simulink model "Simscape_Benchmark_SIM1"  (R2021a)
settings: Solver=ode45  StartTime=0.0  StopTime=PHASE.Ttotal  FixedStep=Benchmark.Sim.Tint  RelTol=1e-5  AbsTol=1e-6
undefined symbols (not defined in the file): Actuators, Analysis, antisym, Benchmark, Bus, Disturbance, FSM, IntialCond, ISOL, K_Coarse_disc_t, Kslew_opt_disc_zoh, Model, MPS, PAYLOAD, PHASE, PMA, RWIsol, RWS, SA, Sensors, Slew, slosh, thr, X, Y, Z
libraries: sm_lib x215, nesl_utility x148, simulink x65, cstblocks x36, sharedtransform x4, vrlib x3, RCTblocks x1
(part 8 of 9)

== system Simscape_Benchmark_SIM1/Dynamical system/Payload System (Telescope structure, FSM, PMA system, Isolator)/Transformation sensors ==
  Mux14 : Mux  Inputs=2
  Mux{15..16,20..21} (4 alike) : Mux  Inputs=3
  Mux22 : Mux  Inputs=2
  PS-Simulink Converter{13..15,40..48} (12 alike) : nesl_utility/PS-Simulink Converter  PhysicalDomain=network_engine_domain  SubClassName=ps_output  LeftPortType=input  RightPortType=output  PseudoPeriodic=off  Frequencies=[]  Unit=inherit  AffineConversion=off
      settings: SourceProductBaseCode=PW,SS
  Transform Sensor4 : sm_lib/Frames and Transforms/Transform Sensor  MeasurementFrame=NonRotatingFollower  SenseAngle=off  SenseAxis=off  SenseAngle1=off  SenseAngle2=off  SenseAngle3=off  SenseQ=off  SenseR=off  SenseOmegaX=off  SenseOmegaY=off  SenseOmegaZ=off  SenseOmega1=off  SenseOmega2=off  SenseOmega3=off  SenseQDot=off  SenseRDot=off  SenseAlphaX=on  SenseAlphaY=on  SenseAlphaZ=on  SenseAlpha1=off  SenseAlpha2=off  SenseAlpha3=off  SenseQDDot=off  SenseRDDot=off  SenseX=off  SenseY=off  SenseZ=off  SenseRad=off  SenseAzim=off  SenseDist=off  SenseInc=off  SenseXDot=off  SenseYDot=off  SenseZDot=off  SenseRadDot=off  SenseAzimDot=off  SenseDistDot=off  SenseIncDot=off  SenseXDDot=on  SenseYDDot=on  SenseZDDot=on  SenseRadDDot=off  SenseAzimDDot=off  SenseDistDDot=off  SenseIncDDot=off
  Transform Sensor7 : sm_lib/Frames and Transforms/Transform Sensor  MeasurementFrame=Base  SenseAngle=off  SenseAxis=off  SenseAngle1=off  SenseAngle2=off  SenseAngle3=off  SenseQ=off  SenseR=off  SenseOmegaX=off  SenseOmegaY=off  SenseOmegaZ=off  SenseOmega1=off  SenseOmega2=off  SenseOmega3=off  SenseQDot=off  SenseRDot=off  SenseAlphaX=on  SenseAlphaY=on  SenseAlphaZ=on  SenseAlpha1=off  SenseAlpha2=off  SenseAlpha3=off  SenseQDDot=off  SenseRDDot=off  SenseX=off  SenseY=off  SenseZ=off  SenseRad=off  SenseAzim=off  SenseDist=off  SenseInc=off  SenseXDot=off  SenseYDot=off  SenseZDot=off  SenseRadDot=off  SenseAzimDot=off  SenseDistDot=off  SenseIncDot=off  SenseXDDot=on  SenseYDDot=on  SenseZDDot=on  SenseRadDDot=off  SenseAzimDDot=off  SenseDistDDot=off  SenseIncDDot=off
  Transform Sensor1 : PMIOPort  Side=Left
  Transform Sensor2 : PMIOPort  Port=2  Side=Left
  xdd_MPC_nonrotating : Outport
  xdd_MPC_Inertial : Outport  Port=2
  wires:
  PS-Simulink Converter45/1 -> Mux15/1
  Mux21/1 -> Mux22/1
  PS-Simulink Converter44/1 -> Mux16/3
  PS-Simulink Converter46/1 -> Mux15/2
  PS-Simulink Converter41/1 -> Mux20/2
  Mux15/1 -> Mux14/2
  PS-Simulink Converter43/1 -> Mux16/2
  Mux14/1 -> xdd_MPC_nonrotating/1
  PS-Simulink Converter48/1 -> Mux20/3
  PS-Simulink Converter47/1 -> Mux15/3
  Mux16/1 -> Mux14/1
  PS-Simulink Converter40/1 -> Mux20/1
  PS-Simulink Converter15/1 -> Mux21/3
  PS-Simulink Converter13/1 -> Mux21/1
  PS-Simulink Converter14/1 -> Mux21/2
  PS-Simulink Converter42/1 -> Mux16/1
  Mux20/1 -> Mux22/2
  Mux22/1 -> xdd_MPC_Inertial/1  "xdd_MPC_Inertial"
  connections:
  Transform Sensor7/RConn1 -- Transform Sensor2/RConn1 -- Transform Sensor4/RConn1
  Transform Sensor4/RConn7 -- PS-Simulink Converter44/LConn1
  Transform Sensor7/LConn1 -- Transform Sensor1/RConn1 -- Transform Sensor4/LConn1
  Transform Sensor4/RConn2 -- PS-Simulink Converter45/LConn1
  Transform Sensor7/RConn6 -- PS-Simulink Converter14/LConn1
  Transform Sensor7/RConn2 -- PS-Simulink Converter40/LConn1
  Transform Sensor4/RConn6 -- PS-Simulink Converter43/LConn1
  Transform Sensor4/RConn3 -- PS-Simulink Converter46/LConn1
  Transform Sensor7/RConn5 -- PS-Simulink Converter13/LConn1
  Transform Sensor4/RConn5 -- PS-Simulink Converter42/LConn1
  Transform Sensor7/RConn3 -- PS-Simulink Converter41/LConn1
  Transform Sensor7/RConn4 -- PS-Simulink Converter48/LConn1
  Transform Sensor7/RConn7 -- PS-Simulink Converter15/LConn1
  Transform Sensor4/RConn4 -- PS-Simulink Converter47/LConn1

== system Simscape_Benchmark_SIM1/Dynamical system/Payload System (Telescope structure, FSM, PMA system, Isolator)/Transformation sensors 2 ==
  Mux13 : Mux  Inputs=2
  Mux2 : Mux  Inputs=3
  Mux3 : Mux  Inputs=3
  PS-Simulink Converter{18..23} (6 alike) : nesl_utility/PS-Simulink Converter  PhysicalDomain=network_engine_domain  SubClassName=ps_output  LeftPortType=input  RightPortType=output  PseudoPeriodic=off  Frequencies=[]  Unit=inherit  AffineConversion=off
      settings: SourceProductBaseCode=PW,SS
  Transform Sensor3 : sm_lib/Frames and Transforms/Transform Sensor  MeasurementFrame=Base  SenseAngle=off  SenseAxis=off  SenseAngle1=off  SenseAngle2=off  SenseAngle3=off  SenseQ=off  SenseR=off  SenseOmegaX=off  SenseOmegaY=off  SenseOmegaZ=off  SenseOmega1=off  SenseOmega2=off  SenseOmega3=off  SenseQDot=off  SenseRDot=off  SenseAlphaX=on  SenseAlphaY=on  SenseAlphaZ=on  SenseAlpha1=off  SenseAlpha2=off  SenseAlpha3=off  SenseQDDot=off  SenseRDDot=off  SenseX=off  SenseY=off  SenseZ=off  SenseRad=off  SenseAzim=off  SenseDist=off  SenseInc=off  SenseXDot=off  SenseYDot=off  SenseZDot=off  SenseRadDot=off  SenseAzimDot=off  SenseDistDot=off  SenseIncDot=off  SenseXDDot=on  SenseYDDot=on  SenseZDDot=on  SenseRadDDot=off  SenseAzimDDot=off  SenseDistDDot=off  SenseIncDDot=off
  Transform Sensor2 : PMIOPort  Side=Left
  Transform Sensor1 : PMIOPort  Port=2  Side=Left
  Out1 : Outport
  wires:
  PS-Simulink Converter19/1 -> Mux3/2
  PS-Simulink Converter18/1 -> Mux3/1
  Mux3/1 -> Mux13/1
  Mux13/1 -> Out1/1
  Mux2/1 -> Mux13/2
  PS-Simulink Converter21/1 -> Mux2/1
  PS-Simulink Converter22/1 -> Mux2/2
  PS-Simulink Converter20/1 -> Mux3/3
  PS-Simulink Converter23/1 -> Mux2/3
  connections:
  PS-Simulink Converter20/LConn1 -- Transform Sensor3/RConn7
  Transform Sensor3/RConn5 -- PS-Simulink Converter18/LConn1
  Transform Sensor3/RConn4 -- PS-Simulink Converter23/LConn1
  Transform Sensor3/RConn3 -- PS-Simulink Converter22/LConn1
  Transform Sensor3/RConn2 -- PS-Simulink Converter21/LConn1
  Transform Sensor3/RConn6 -- PS-Simulink Converter19/LConn1
  Transform Sensor2/RConn1 -- Transform Sensor3/LConn1
  Transform Sensor3/RConn1 -- Transform Sensor1/RConn1

== system Simscape_Benchmark_SIM1/Dynamical system/RCS models/RCS (thruster model) ==
  Cmd_force : Inport  PortDimensions=3
  Cmd_Torque : Inport  Port=2  PortDimensions=3
  Allocation Function (Updated) : MATLABFcn  MATLABFcn=Thr_AllocationFunct  OutputDimensions=thr.nb_thr+1
  Clock : Clock
  Constant : Constant  Value=thr.sc_thrust_Ht
  Constant1 : Constant  Value=thr.F
  Constant10 : Constant  Value=thr.sc_thrust_Ht_reshaped'
  Constant11 : Constant  Value=thr.nb_thr
  Constant13 : Constant  Value=thr.F
  Constant2 : Constant  Value=thr.sc_thrust_Hf
  Constant3 : Constant  Value=thr.nb_thr
  Constant4 : Constant  Value=Model.ACS_sampling.Ts
  Constant6 : Constant  Value=thr.u_min
  Constant8 : Constant  Value=zeros(thr.nb_thr,1)
  Constant9 : Constant  Value=thr.sc_thrust_Hf_reshaped'
  Demux1 : Demux  Outputs=[thr.nb_thr,1]
  Demux2 : Demux  Outputs=[3,3]
  Gain : Gain  Gain=thr.F
  Gain1 : Gain  Gain=thr.F
  Gain2 : Gain  Gain=thr.F
  MATLAB Function1 : MATLAB Function  TreatAsAtomicUnit=on  SystemSampleTime=thr.MIB_time
  Matrix Concatenate : Concatenate  Mode=Multidimensional array
  Mux : Mux  Inputs=2
  Mux2 : Mux  Inputs=2
  Mux3 : Mux  Inputs=[6,1,1,thr.nb_thr*3,thr.nb_thr*3]
  Product : Product  Multiplication=Matrix(*)
  Scope1 : Scope  NumInputPorts=2
  Scope2 : Scope
  Sum : Sum  Inputs=-+
  Thruster dynamic response (2nd order) : cstblocks/LTI System  Commented=through  sys=tf(thr.om^2,[1 2*thr.damp*thr.om thr.om^2])*eye(thr.nb_thr)  IC=[]
  Thr_Force : Outport
  Thr_Force_NoPWM : Outport  Port=2
  Thr_activated : Outport  Port=3
  wires:
  Constant10/1 -> Mux3/5  "thr.nb_thr*3"
  Constant9/1 -> Mux3/4  "thr.nb_thr*3"
  Constant2/1 -> Matrix Concatenate/1
  Constant1/1 -> MATLAB Function1/2(u_thr)
  Constant8/1 -> MATLAB Function1/7(y_size)
  Constant3/1 -> MATLAB Function1/5(nb_thr)
  Mux2/1 -> Mux3/1, Sum/1
  Constant4/1 -> MATLAB Function1/3(Sampling_time)
  Sum/1 -> Scope2/1
  Constant/1 -> Matrix Concatenate/2
  Constant13/1 -> Mux3/3  "1"
  Demux1/1 -> Mux/2, Gain2/1, Gain/1, Product/2  "U_cont"
  Demux1/2 -> Thr_activated/1  "n_activated"
  Constant6/1 -> MATLAB Function1/4(u_min)
  Matrix Concatenate/1 -> Product/1
  Mux3/1 -> Mux/1
  Allocation Function (Updated)/1 -> Demux1/1
  Constant11/1 -> Mux3/2  "1"
  Cmd_force/1 -> Mux2/1
  Cmd_Torque/1 -> Mux2/2
  MATLAB Function1/1(y) -> Thruster dynamic response (2nd order)/1
  Clock/1 -> MATLAB Function1/6(Time)
  Demux2/1 -> Scope1/1
  Product/1 -> Sum/2, Gain1/1
  Demux2/2 -> Scope1/2
  Gain/1 -> Thr_Force_NoPWM/1
  Gain1/1 -> Demux2/1
  Mux/1 -> Allocation Function (Updated)/1
  Thruster dynamic response (2nd order)/1 -> Thr_Force/1
  Gain2/1 -> MATLAB Function1/1(U_cont)

== system Simscape_Benchmark_SIM1/Dynamical system/WEMS + Reaction wheels/Friction compensation filter ==
  speed : Inport
  torque : Inport  Port=2
  Enable : EnablePort
  1/Ts : Gain  Gain=1/Model.ACS_sampling.Ts
  Clock : Clock
  Constant : Constant  Value=0
  Constant1 : Constant  Value=[0;0;0;0]
  Delay1 : Delay  DelayLength=1  InitialConditionSource=Input port  InitialCondition=RWS.w1simscape
      settings: InputPortMap=u0,p4
  Delay2 : Delay  DelayLength=1  InitialConditionSource=Input port  InitialCondition=RWS.w2simscape
      settings: InputPortMap=u0,p4
  Delay3 : Delay  DelayLength=1  InitialCondition=0
  Delay4 : Delay  DelayLength=1  InitialConditionSource=Input port  InitialCondition=RWS.w3simscape
      settings: InputPortMap=u0,p4
  Delay5 : Delay  DelayLength=1  InitialConditionSource=Input port  InitialCondition=RWS.w4simscape
      settings: InputPortMap=u0,p4
  Demux6 : Demux
  I_wheel : Gain  Gain=RWS.Iw
  InitialCond_1 : Constant  Value=RWS.w1simscape
  InitialCond_2 : Constant  Value=RWS.w2simscape
  InitialCond_3 : Constant  Value=RWS.w3simscape
  InitialCond_4 : Constant  Value=RWS.w4simscape
  LTI System1 : cstblocks/LTI System  sys=RWS.FrictionEstimation.FilterD  IC=0
  Mux4 : Mux
  RWS.FrictionEstimation.T_excludeTransient : Constant  Value=RWS.FrictionEstimation.T_excludeTransient
  Rate Transition : RateTransition  OutPortSampleTime=Model.ACS_sampling.Ts
  Sum : Sum  Inputs=|+-
  Sum1 : Sum  Inputs=+|-
  Sum2 : Sum  Inputs=|+-
  Switch : Switch  Criteria=u2 > Threshold
  Terminator : Terminator
  Out1 : Outport  InitialOutput=[0;0;0;0]
  wires:
  Sum1/1 -> LTI System1/1
  Demux6/1 -> Delay1/1
  Constant1/1 -> Switch/3
  Delay4/1 -> Mux4/3
  Clock/1 -> Sum2/1
  Delay3/1 -> Sum1/2
  LTI System1/1 -> Switch/1
  Sum/1 -> I_wheel/1
  Switch/1 -> Out1/1  "estimated"
  Demux6/3 -> Delay4/1
  Delay2/1 -> Mux4/2
  torque/1 -> Delay3/1
  Demux6/4 -> Delay5/1
  speed/1 -> Sum/1, Demux6/1
  Delay5/1 -> Mux4/4
  Mux4/1 -> Sum/2
  Demux6/2 -> Delay2/1
  1/Ts/1 -> Sum1/1
  Rate Transition/1 -> Switch/2
  Delay1/1 -> Mux4/1
  Constant/1 -> Sum2/2
  Sum2/1 -> Rate Transition/1
  RWS.FrictionEstimation.T_excludeTransient/1 -> Terminator/1
  I_wheel/1 -> 1/Ts/1
  InitialCond_1/1 -> Delay1/2
  InitialCond_2/1 -> Delay2/2
  InitialCond_3/1 -> Delay4/2
  InitialCond_4/1 -> Delay5/2

== system Simscape_Benchmark_SIM1/Dynamical system/WEMS + Reaction wheels/RW saturation and friction model ==
  note: 1) Add Subsystem or Model blocks as valid variant choices.
      | 2) You cannot connect blocks at this level. At simulation, connectivity is automatically
      | determined, based on the active variant and port name matching.
  In1 : Inport
  No saturations - No friction model : Subsystem  VariantControl=Benchmark.config.status.RWS_Sat==0 && Benchmark.config.status.RWS_Fric==0 && Benchmark.config.status.RWS_Frict_spikes==0
  Saturations +  friction model : Subsystem  VariantControl=Benchmark.config.status.RWS_Sat==1 && Benchmark.config.status.RWS_Fric==1 && Benchmark.config.status.RWS_Frict_spikes==0
  Saturations + friction model + friction spikes : Subsystem  VariantControl=Benchmark.config.status.RWS_Sat==1 && Benchmark.config.status.RWS_Fric==1 && Benchmark.config.status.RWS_Frict_spikes==1
  Saturations - No friction model : Subsystem  VariantControl=Benchmark.config.status.RWS_Sat==1 && Benchmark.config.status.RWS_Fric==0 && Benchmark.config.status.RWS_Frict_spikes==0
  Out1 : Outport

== system Simscape_Benchmark_SIM1/Dynamical system/WEMS + Reaction wheels/Reaction wheel Mass//inertia (balanced and unbalanced model) ==
  Balanced RWS : Subsystem  VariantControl="Benchmark.config.status.RWS_Harmdist==   0"
  RWS with disturbance harmonics : Subsystem  VariantControl="Benchmark.config.status.RWS_Harmdist==   1"
  Connection Port : PMIOPort  Tag=PMCPort  Side=Left
  Connection Port1 : PMIOPort  Tag=PMCPort  Port=2  Side=Left
  Connection Port2 : PMIOPort  Tag=PMCPort  Port=3  Side=Left
  Connection Port3 : PMIOPort  Tag=PMCPort  Port=4  Side=Left

== system Simscape_Benchmark_SIM1/Sensors/Accelerometer Mirror 1/acc_M1 ==
  note: Constant PSD such that
      | its integral (from 0 to Nyquist frequency) is 1
  note: After scaling: One-sided PSD with value equal to 1
      | up to Nyquist frequency
  Gain : Gain
  Gain1 : Gain  Gain=sqrt(0.5/Sensors.ACCm1.SampleTime)
  Gain2 : Gain  Gain=sqrt(0.5/Sensors.ACCm1.SampleTime)
  Gain3 : Gain
  Gain4 : Gain
  Gain7 : Gain  Gain=sqrt(0.5/Sensors.ACCm1.SampleTime)
  Mux : Mux  Inputs=6
  Noise_accM1_rotx : simulink/Sources/Band-Limited White Noise  Cov=Sensors.ACCm1.NoiseProtx  Ts=Sensors.ACCm1.SampleTime  seed=Sensors.ACCm1.Seed(4)
  Noise_accM1_roty : simulink/Sources/Band-Limited White Noise  Cov=Sensors.ACCm1.NoiseProty  Ts=Sensors.ACCm1.SampleTime  seed=Sensors.ACCm1.Seed(5)
  Noise_accM1_rotz : simulink/Sources/Band-Limited White Noise  Cov=Sensors.ACCm1.NoiseProtz  Ts=Sensors.ACCm1.SampleTime  seed=Sensors.ACCm1.Seed(6)
  Noise_accM1_x : simulink/Sources/Band-Limited White Noise  Cov=Sensors.ACCm1.NoisePx  Ts=Sensors.ACCm1.SampleTime  seed=Sensors.ACCm1.Seed(1)
  Noise_accM1_y : simulink/Sources/Band-Limited White Noise  Cov=Sensors.ACCm1.NoisePy  Ts=Sensors.ACCm1.SampleTime  seed=Sensors.ACCm1.Seed(2)
  Noise_accM1_z : simulink/Sources/Band-Limited White Noise  Cov=Sensors.ACCm1.NoisePz  Ts=Sensors.ACCm1.SampleTime  seed=Sensors.ACCm1.Seed(3)
  Sensors.ACCm1.NoisePxFilter : cstblocks/LTI System  sys=Sensors.ACCm1.NoisePxFilter  IC=[]
  Sensors.ACCm1.NoisePyFilter : cstblocks/LTI System  sys=Sensors.ACCm1.NoisePyFilter  IC=[]
  Sensors.ACCm1.NoisePzFilter : cstblocks/LTI System  sys=Sensors.ACCm1.NoisePzFilter  IC=[]
  Out1 : Outport
  wires:
  Sensors.ACCm1.NoisePxFilter/1 -> Mux/1
  Mux/1 -> Out1/1
  Gain1/1 -> Sensors.ACCm1.NoisePyFilter/1
  Gain7/1 -> Sensors.ACCm1.NoisePxFilter/1
  Sensors.ACCm1.NoisePyFilter/1 -> Mux/2
  Sensors.ACCm1.NoisePzFilter/1 -> Mux/3
  Noise_accM1_rotx/1 -> Gain/1
  Noise_accM1_roty/1 -> Gain3/1
  Noise_accM1_rotz/1 -> Gain4/1
  Noise_accM1_x/1 -> Gain7/1
  Noise_accM1_y/1 -> Gain1/1
  Noise_accM1_z/1 -> Gain2/1
  Gain2/1 -> Sensors.ACCm1.NoisePzFilter/1
  Gain/1 -> Mux/4
  Gain3/1 -> Mux/5
  Gain4/1 -> Mux/6

== system Simscape_Benchmark_SIM1/Sensors/Accelerometer Mirror 2/acc_M2 ==
  Gain1 : Gain  Gain=sqrt(0.5/Sensors.ACCm2.SampleTime)
  Gain2 : Gain  Gain=sqrt(0.5/Sensors.ACCm2.SampleTime)
  Gain3 : Gain
  Gain4 : Gain
  Gain5 : Gain
  Gain7 : Gain  Gain=sqrt(0.5/Sensors.ACCm2.SampleTime)
  Mux : Mux  Inputs=6
  Noise_accM2_rotx : simulink/Sources/Band-Limited White Noise  Cov=Sensors.ACCm2.NoiseProtx  Ts=Sensors.ACCm2.SampleTime  seed=Sensors.ACCm2.Seed(4)
  Noise_accM2_roty : simulink/Sources/Band-Limited White Noise  Cov=Sensors.ACCm2.NoiseProty  Ts=Sensors.ACCm2.SampleTime  seed=Sensors.ACCm2.Seed(5)
  Noise_accM2_rotz : simulink/Sources/Band-Limited White Noise  Cov=Sensors.ACCm2.NoiseProtz  Ts=Sensors.ACCm2.SampleTime  seed=Sensors.ACCm2.Seed(6)
  Noise_accM2_x : simulink/Sources/Band-Limited White Noise  Cov=Sensors.ACCm2.NoisePx  Ts=Sensors.ACCm2.SampleTime  seed=Sensors.ACCm2.Seed(1)
  Noise_accM2_y : simulink/Sources/Band-Limited White Noise  Cov=Sensors.ACCm2.NoisePy  Ts=Sensors.ACCm2.SampleTime  seed=Sensors.ACCm2.Seed(2)
  Noise_accM2_z : simulink/Sources/Band-Limited White Noise  Cov=Sensors.ACCm2.NoisePz  Ts=Sensors.ACCm2.SampleTime  seed=Sensors.ACCm2.Seed(3)
  Sensors.ACCm2.NoisePxFilter : cstblocks/LTI System  sys=Sensors.ACCm2.NoisePxFilter  IC=[]
  Sensors.ACCm2.NoisePyFilter : cstblocks/LTI System  sys=Sensors.ACCm2.NoisePyFilter  IC=[]
  Sensors.ACCm2.NoisePzFilter : cstblocks/LTI System  sys=Sensors.ACCm2.NoisePzFilter  IC=[]
  Out1 : Outport
  wires:
  Sensors.ACCm2.NoisePxFilter/1 -> Mux/1
  Mux/1 -> Out1/1
  Gain1/1 -> Sensors.ACCm2.NoisePyFilter/1
  Gain2/1 -> Sensors.ACCm2.NoisePzFilter/1
  Gain7/1 -> Sensors.ACCm2.NoisePxFilter/1
  Sensors.ACCm2.NoisePyFilter/1 -> Mux/2
  Sensors.ACCm2.NoisePzFilter/1 -> Mux/3
  Noise_accM2_rotz/1 -> Gain5/1
  Gain3/1 -> Mux/4
  Gain4/1 -> Mux/5
  Noise_accM2_z/1 -> Gain2/1
  Noise_accM2_y/1 -> Gain1/1
  Noise_accM2_x/1 -> Gain7/1
  Noise_accM2_rotx/1 -> Gain3/1
  Noise_accM2_roty/1 -> Gain4/1
  Gain5/1 -> Mux/6

== system Simscape_Benchmark_SIM1/Sensors/Accelerometer at detector/acc_dect ==
  Gain1 : Gain  Gain=sqrt(0.5/Sensors.ACCdect.SampleTime)
  Gain2 : Gain  Gain=sqrt(0.5/Sensors.ACCdect.SampleTime)
  Gain3 : Gain
  Gain4 : Gain
  Gain5 : Gain
  Gain7 : Gain  Gain=sqrt(0.5/Sensors.ACCdect.SampleTime)
  Mux : Mux  Inputs=6
  Noise_accdect_rotx : simulink/Sources/Band-Limited White Noise  Cov=Sensors.ACCdect.NoiseProtx  Ts=Sensors.ACCdect.SampleTime  seed=Sensors.ACCdect.Seed(4)
  Noise_accdect_roty : simulink/Sources/Band-Limited White Noise  Cov=Sensors.ACCdect.NoiseProty  Ts=Sensors.ACCdect.SampleTime  seed=Sensors.ACCdect.Seed(5)
  Noise_accdect_rotz : simulink/Sources/Band-Limited White Noise  Cov=Sensors.ACCdect.NoiseProtz  Ts=Sensors.ACCdect.SampleTime  seed=Sensors.ACCdect.Seed(6)
  Noise_accdect_x : simulink/Sources/Band-Limited White Noise  Cov=Sensors.ACCdect.NoisePx  Ts=Sensors.ACCdect.SampleTime  seed=Sensors.ACCdect.Seed(1)
  Noise_accdect_y : simulink/Sources/Band-Limited White Noise  Cov=Sensors.ACCdect.NoisePy  Ts=Sensors.ACCdect.SampleTime  seed=Sensors.ACCdect.Seed(2)
  Noise_accdect_z : simulink/Sources/Band-Limited White Noise  Cov=Sensors.ACCdect.NoisePz  Ts=Sensors.ACCdect.SampleTime  seed=Sensors.ACCdect.Seed(3)
  Sensors.ACCdect.NoisePxFilter : cstblocks/LTI System  sys=Sensors.ACCm2.NoisePxFilter  IC=[]
  Sensors.ACCdect.NoisePyFilter : cstblocks/LTI System  sys=Sensors.ACCm2.NoisePyFilter  IC=[]
  Sensors.ACCdect.NoisePzFilter : cstblocks/LTI System  sys=Sensors.ACCm2.NoisePzFilter  IC=[]
  Out1 : Outport
  wires:
  Sensors.ACCdect.NoisePxFilter/1 -> Mux/1
  Mux/1 -> Out1/1
  Sensors.ACCdect.NoisePyFilter/1 -> Mux/2
  Sensors.ACCdect.NoisePzFilter/1 -> Mux/3
  Gain5/1 -> Mux/6
  Gain4/1 -> Mux/4
  Gain3/1 -> Mux/5
  Noise_accdect_x/1 -> Gain7/1
  Gain7/1 -> Sensors.ACCdect.NoisePxFilter/1
  Noise_accdect_y/1 -> Gain1/1
  Gain1/1 -> Sensors.ACCdect.NoisePyFilter/1
  Gain2/1 -> Sensors.ACCdect.NoisePzFilter/1
  Noise_accdect_z/1 -> Gain2/1
  Noise_accdect_rotx/1 -> Gain4/1
  Noise_accdect_roty/1 -> Gain3/1
  Noise_accdect_rotz/1 -> Gain5/1

== system Simscape_Benchmark_SIM1/Sensors/Fine Guidance Sensor (FGS)/FGS noise ==
  Mux : Mux  Inputs=2
  Noise_fgs_x : simulink/Sources/Band-Limited White Noise  Cov=Sensors.FGS.NoisePx  Ts=Sensors.FGS.SampleTime  seed=Sensors.FGS.Seed(1)
  noise_fgs_y : simulink/Sources/Band-Limited White Noise  Cov=Sensors.FGS.NoisePy  Ts=Sensors.FGS.SampleTime  seed=Sensors.FGS.Seed(2)
  Out1 : Outport
  wires:
  Noise_fgs_x/1 -> Mux/1
  Mux/1 -> Out1/1
  noise_fgs_y/1 -> Mux/2

== system Simscape_Benchmark_SIM1/Sensors/Gyro (Coarse//fine)/Noise - Corse gyro ==
  ARW_1 : simulink/Sources/Band-Limited White Noise  Cov=Sensors.GYROc.ARW_NoisePx  Ts=Sensors.GYROc.SampleTime  seed=Sensors.GYROc.ARW_Seed(1)
  ARW_2 : simulink/Sources/Band-Limited White Noise  Cov=Sensors.GYROc.ARW_NoisePy  Ts=Sensors.GYROc.SampleTime  seed=Sensors.GYROc.ARW_Seed(2)
  ARW_3 : simulink/Sources/Band-Limited White Noise  Cov=Sensors.GYROc.ARW_NoisePz  Ts=Sensors.GYROc.SampleTime  seed=Sensors.GYROc.ARW_Seed(3)
  BiasInstability_1 : simulink/Sources/Band-Limited White Noise  Cov=Sensors.GYROc.SampleTime  Ts=Sensors.GYROc.SampleTime  seed=Sensors.GYROf.BiasInstability(1)
  BiasInstability_2 : simulink/Sources/Band-Limited White Noise  Cov=Sensors.GYROc.SampleTime  Ts=Sensors.GYROc.SampleTime  seed=Sensors.GYROf.BiasInstability(2)
  BiasInstability_3 : simulink/Sources/Band-Limited White Noise  Cov=Sensors.GYROc.SampleTime  Ts=Sensors.GYROc.SampleTime  seed=Sensors.GYROf.BiasInstability(3)
  Gain1 : Gain  Gain=sqrt(0.5/Sensors.GYROc.SampleTime)
  Gain2 : Gain  Gain=sqrt(0.5/Sensors.GYROc.SampleTime)
  Gain7 : Gain  Gain=sqrt(0.5/Sensors.GYROc.SampleTime)
  LTI System1 : cstblocks/LTI System  sys=Sensors.GYROc.FlickerDisc  IC=[]
  LTI System2 : cstblocks/LTI System  sys=Sensors.GYROc.FlickerDisc  IC=[]
  LTI System3 : cstblocks/LTI System  sys=Sensors.GYROc.FlickerDisc  IC=[]
  Mux : Mux  Inputs=3
  Sensors.GYROc.BiasInstability_SelectSim : Gain  Gain=Sensors.GYROc.BiasInstability_SelectSim
  Sensors.GYROc.BiasInstability_SelectSim2 : Gain  Gain=Sensors.GYROc.BiasInstability_SelectSim
  Sensors.GYROc.BiasInstability_SelectSim3 : Gain  Gain=Sensors.GYROc.BiasInstability_SelectSim
  Sum1 : Sum
  Sum2 : Sum
  Sum3 : Sum
  Out1 : Outport
  wires:
  Sum2/1 -> Mux/2
  ARW_1/1 -> Sum1/1
  Mux/1 -> Out1/1
  Sum3/1 -> Mux/3
  Sum1/1 -> Mux/1
  ARW_2/1 -> Sum2/1
  ARW_3/1 -> Sum3/1
  LTI System2/1 -> Sensors.GYROc.BiasInstability_SelectSim2/1
  LTI System3/1 -> Sensors.GYROc.BiasInstability_SelectSim3/1
  BiasInstability_1/1 -> Gain7/1
  LTI System1/1 -> Sensors.GYROc.BiasInstability_SelectSim/1
  Sensors.GYROc.BiasInstability_SelectSim2/1 -> Sum2/2
  Sensors.GYROc.BiasInstability_SelectSim/1 -> Sum1/2
  Sensors.GYROc.BiasInstability_SelectSim3/1 -> Sum3/2
  Gain7/1 -> LTI System1/1
  Gain1/1 -> LTI System2/1
  BiasInstability_2/1 -> Gain1/1
  Gain2/1 -> LTI System3/1
  BiasInstability_3/1 -> Gain2/1

== system Simscape_Benchmark_SIM1/Sensors/Gyro (Coarse//fine)/Noise Fine Gyro ==
  ARW_1 : simulink/Sources/Band-Limited White Noise  Cov=Sensors.GYROf.ARW_NoisePx  Ts=Sensors.GYROf.SampleTime  seed=Sensors.GYROf.ARW_Seed(1)
  ARW_2 : simulink/Sources/Band-Limited White Noise  Cov=Sensors.GYROf.ARW_NoisePy  Ts=Sensors.GYROf.SampleTime  seed=Sensors.GYROf.ARW_Seed(2)
  ARW_3 : simulink/Sources/Band-Limited White Noise  Cov=Sensors.GYROf.ARW_NoisePz  Ts=Sensors.GYROf.SampleTime  seed=Sensors.GYROf.ARW_Seed(3)
  BiasInstability_1 : simulink/Sources/Band-Limited White Noise  Cov=Sensors.GYROf.SampleTime  Ts=Sensors.GYROf.SampleTime  seed=Sensors.GYROf.BiasInstability(1)
  BiasInstability_2 : simulink/Sources/Band-Limited White Noise  Cov=Sensors.GYROf.SampleTime  Ts=Sensors.GYROf.SampleTime  seed=Sensors.GYROf.BiasInstability(2)
  BiasInstability_3 : simulink/Sources/Band-Limited White Noise  Cov=Sensors.GYROf.SampleTime  Ts=Sensors.GYROf.SampleTime  seed=Sensors.GYROf.BiasInstability(3)
  Gain1 : Gain  Gain=sqrt(0.5/Sensors.GYROf.SampleTime)
  Gain2 : Gain  Gain=sqrt(0.5/Sensors.GYROf.SampleTime)
  Gain7 : Gain  Gain=sqrt(0.5/Sensors.GYROf.SampleTime)
  LTI System1 : cstblocks/LTI System  sys=Sensors.GYROf.FlickerDisc  IC=[]
  LTI System2 : cstblocks/LTI System  sys=Sensors.GYROf.FlickerDisc  IC=[]
  LTI System3 : cstblocks/LTI System  sys=Sensors.GYROf.FlickerDisc  IC=[]
  Mux : Mux  Inputs=3
  Sensors.GYROf.BiasInstability_SelectSim : Gain  Gain=Sensors.GYROf.BiasInstability_SelectSim
  Sensors.GYROf.BiasInstability_SelectSim1 : Gain  Gain=Sensors.GYROf.BiasInstability_SelectSim
  Sensors.GYROf.BiasInstability_SelectSim2 : Gain  Gain=Sensors.GYROf.BiasInstability_SelectSim
  Sum1 : Sum
  Sum2 : Sum
  Sum3 : Sum
  Out1 : Outport
  wires:
  ARW_2/1 -> Sum2/1
  ARW_3/1 -> Sum3/1
  Sum3/1 -> Mux/3
  ARW_1/1 -> Sum1/1
  Sensors.GYROf.BiasInstability_SelectSim/1 -> Sum1/2
  Sensors.GYROf.BiasInstability_SelectSim1/1 -> Sum2/2
  Mux/1 -> Out1/1
  Sum1/1 -> Mux/1
  Sum2/1 -> Mux/2
  Sensors.GYROf.BiasInstability_SelectSim2/1 -> Sum3/2
  LTI System1/1 -> Sensors.GYROf.BiasInstability_SelectSim/1
  Gain7/1 -> LTI System1/1
  Gain1/1 -> LTI System2/1
  LTI System2/1 -> Sensors.GYROf.BiasInstability_SelectSim1/1
  LTI System3/1 -> Sensors.GYROf.BiasInstability_SelectSim2/1
  BiasInstability_1/1 -> Gain7/1
  BiasInstability_2/1 -> Gain1/1
  BiasInstability_3/1 -> Gain2/1
  Gain2/1 -> LTI System3/1

== system Simscape_Benchmark_SIM1/Sensors/RW tachometer/RW speed measurement noise ==
  Mux : Mux
  Noise_RW_1 : simulink/Sources/Band-Limited White Noise  Cov=Sensors.RW_tachometer.Noise  Ts=Sensors.RW_tachometer.SampleTime  seed=Sensors.RW_tachometer.Seed(1)
  Noise_RW_2 : simulink/Sources/Band-Limited White Noise  Cov=Sensors.RW_tachometer.Noise  Ts=Sensors.RW_tachometer.SampleTime  seed=Sensors.RW_tachometer.Seed(2)
  Noise_RW_3 : simulink/Sources/Band-Limited White Noise  Cov=Sensors.RW_tachometer.Noise  Ts=Sensors.RW_tachometer.SampleTime  seed=Sensors.RW_tachometer.Seed(3)
  Noise_RW_4 : simulink/Sources/Band-Limited White Noise  Cov=Sensors.RW_tachometer.Noise  Ts=Sensors.RW_tachometer.SampleTime  seed=Sensors.RW_tachometer.Seed(4)
  Out1 : Outport
  wires:
  Noise_RW_1/1 -> Mux/1
  Mux/1 -> Out1/1
  Noise_RW_2/1 -> Mux/2
  Noise_RW_4/1 -> Mux/4
  Noise_RW_3/1 -> Mux/3

== system Simscape_Benchmark_SIM1/Sensors/Rotation measurements of the fast steering mirror (FSM)/FGS noise ==
  Mux : Mux  Inputs=2
  Noise_fsm_rotx : simulink/Sources/Band-Limited White Noise  Cov=Sensors.FSM.NoiseProtx  Ts=Sensors.FSM.SampleTime  seed=Sensors.FSM.Seed(1)
  Noise_fsm_roty : simulink/Sources/Band-Limited White Noise  Cov=Sensors.FSM.NoiseProty  Ts=Sensors.FSM.SampleTime  seed=Sensors.FSM.Seed(2)
  Out1 : Outport
  wires:
  Noise_fsm_rotx/1 -> Mux/1
  Mux/1 -> Out1/1
  Noise_fsm_roty/1 -> Mux/2

== system Simscape_Benchmark_SIM1/Sensors/Star tracker/SST noise ==
  Band-Limited White Noise : simulink/Sources/Band-Limited White Noise  Cov=Sensors.SST.NoisePx  Ts=Sensors.SST.SampleTime  seed=Sensors.SST.Seed(1)
  Band-Limited White Noise1 : simulink/Sources/Band-Limited White Noise  Cov=Sensors.SST.NoisePy  Ts=Sensors.SST.SampleTime  seed=Sensors.SST.Seed(2)
  Band-Limited White Noise2 : simulink/Sources/Band-Limited White Noise  Cov=Sensors.SST.NoisePz  Ts=Sensors.SST.SampleTime  seed=Sensors.SST.Seed(3)
  Constant : Constant  Value=Sensors.SST.biasx  SampleTime=Sensors.SST.SampleTime
  Constant1 : Constant  Value=Sensors.SST.biasy  SampleTime=Sensors.SST.SampleTime
  Constant2 : Constant  Value=Sensors.SST.biasz  SampleTime=Sensors.SST.SampleTime
  Mux : Mux  Inputs=3
  Random Number : RandomNumber  Commented=on  Mean=Sensors.SST.Mean  Variance=Sensors.SST.VarianceX  Seed=Sensors.SST.Seed(1)  SampleTime=Sensors.SST.SampleTime
  Random Number1 : RandomNumber  Commented=on  Mean=Sensors.SST.Mean  Variance=Sensors.SST.VarianceY  Seed=Sensors.SST.Seed(2)  SampleTime=Sensors.SST.SampleTime
  Random Number2 : RandomNumber  Commented=on  Mean=Sensors.SST.Mean  Variance=Sensors.SST.VarianceZ  Seed=Sensors.SST.Seed(3)  SampleTime=Sensors.SST.SampleTime
  Sum : Sum  Inputs=++|
  Sum1 : Sum  Inputs=++|
  Sum2 : Sum  Inputs=++|
  Out1 : Outport
  wires:
  Band-Limited White Noise/1 -> Sum/2
  Mux/1 -> Out1/1
  Band-Limited White Noise1/1 -> Sum1/2
  Band-Limited White Noise2/1 -> Sum2/2
  Sum/1 -> Mux/1
  Constant/1 -> Sum/1
  Sum1/1 -> Mux/2
  Constant1/1 -> Sum1/1
  Sum2/1 -> Mux/3
  Constant2/1 -> Sum2/1

== system Simscape_Benchmark_SIM1/Dynamical system/Payload System (Telescope structure, FSM, PMA system, Isolator)/Integration/Quaternion Integration2 ==
  om : Inport
  Q_init : Inport  Port=2
  Integrator6 : Integrator  InitialConditionSource=external
  Subsystem : Subsystem
  q_4 : Outport
  wires:
  Subsystem/1(Out1) -> Integrator6/1
  om/1 -> Subsystem/2(om)
  Integrator6/1 -> q_4/1, Subsystem/1(q_4)
  Q_init/1 -> Integrator6/2

== system Simscape_Benchmark_SIM1/Dynamical system/Payload System (Telescope structure, FSM, PMA system, Isolator)/Integration 1/Quaternion Integration1 ==
  om : Inport
  Q_init : Inport  Port=2
  Integrator6 : Integrator  InitialConditionSource=external
  Subsystem : Subsystem
  q_4 : Outport
  wires:
  Subsystem/1(Out1) -> Integrator6/1
  om/1 -> Subsystem/2(om)
  Integrator6/1 -> q_4/1, Subsystem/1(q_4)
  Q_init/1 -> Integrator6/2

== system Simscape_Benchmark_SIM1/Dynamical system/Payload System (Telescope structure, FSM, PMA system, Isolator)/Quaternion Integration/Subsystem ==
  q_4 : Inport
  om : Inport  Port=2
  Cross Product : vrlib/Utilities/Cross Product
  Demux : Demux  Outputs=[1 3]
  Dot Product : DotProduct  InputSameDT=on  OutDataTypeStr=Inherit: Inherit via internal rule
  Gain : Gain  Gain=0.5
  Gain1 : Gain  Gain=-1
  Gain2 : Gain  Gain=-1
  Mux : Mux  Inputs=[1,3]
  Product : Product
  Sum : Sum  Inputs=|+-
  Out1 : Outport
  wires:
  Gain/1 -> Out1/1
  Mux/1 -> Gain/1
  Demux/1 -> Product/2  "q0"
  Demux/2 -> Cross Product/2, Dot Product/2  "q"
  q_4/1 -> Demux/1
  Dot Product/1 -> Gain1/1
  om/1 -> Cross Product/1, Product/1, Dot Product/1
  Gain1/1 -> Mux/1
  Sum/1 -> Mux/2
  Product/1 -> Sum/1
  Cross Product/1 -> Gain2/1
  Gain2/1 -> Sum/2

== system Simscape_Benchmark_SIM1/Dynamical system/WEMS + Reaction wheels/RW saturation and friction model/No saturations - No friction model ==
  In1 : Inport
  Out1 : Outport
  wires:
  In1/1 -> Out1/1

== system Simscape_Benchmark_SIM1/Dynamical system/WEMS + Reaction wheels/RW saturation and friction model/Saturations +  friction model ==
  In1 : Inport
  RW friction model : Subsystem
  Terminator2 : Terminator
  sat_max_torque : Saturate  UpperLimit=RWS.max_torque  LowerLimit=-RWS.max_torque
  Out1 : Outport
  wires:
  In1/1 -> sat_max_torque/1
  sat_max_torque/1 -> RW friction model/1(Trq_cmd_rw)
  RW friction model/1(Torque_RW) -> Out1/1
  RW friction model/2(RW_TRQfriction) -> Terminator2/1

== system Simscape_Benchmark_SIM1/Dynamical system/WEMS + Reaction wheels/RW saturation and friction model/Saturations + friction model + friction spikes ==
  In1 : Inport
  Gain : Gain  Gain=-1
  Mux : Mux
  Product : Product
  RW friction model : Subsystem
  Rate Transition : RateTransition  OutPortSampleTime=Model.ACS_sampling.Ts
  Spike generation RW1 : Subsystem
  Spike generation RW2 : Subsystem
  Spike generation RW3 : Subsystem
  Spike generation RW4 : Subsystem
  Sum : Sum
  Terminator2 : Terminator
  sat_max_torque : Saturate  UpperLimit=RWS.max_torque  LowerLimit=-RWS.max_torque
  Out1 : Outport
  tag scope: RW_torque_spikes=global
  wires:
  In1/1 -> sat_max_torque/1
  Sum/1 -> Out1/1
  Mux/1 -> Rate Transition/1
  RW friction model/1(Torque_RW) -> Sum/1
  RW friction model/2(RW_TRQfriction) -> Terminator2/1
  sat_max_torque/1 -> RW friction model/1(Trq_cmd_rw)
  Spike generation RW1/1(Out1) -> Mux/1
  Spike generation RW3/1(Out1) -> Mux/3
  Spike generation RW2/1(Out1) -> Mux/2
  Spike generation RW4/1(Out1) -> Mux/4
  RW friction model/3(sign_omega) -> Product/1
  Rate Transition/1 -> Gain/1
  Product/1 -> [RW_torque_spikes], Sum/2
  Gain/1 -> Product/2

== system Simscape_Benchmark_SIM1/Dynamical system/WEMS + Reaction wheels/RW saturation and friction model/Saturations - No friction model ==
  In1 : Inport
  sat_max_torque : Saturate  UpperLimit=RWS.max_torque  LowerLimit=-RWS.max_torque
  Out1 : Outport
  wires:
  In1/1 -> sat_max_torque/1
  sat_max_torque/1 -> Out1/1

== system Simscape_Benchmark_SIM1/Dynamical system/WEMS + Reaction wheels/Reaction wheel Mass//inertia (balanced and unbalanced model)/Balanced RWS ==
  Cylindrical Solid{,1..3} (4 alike) : sm_lib/Body Elements/Cylindrical Solid  GraphicAmbientColor=[0.15 0.15 0.15 1.0]  BasedOnType=Density  CenterOfMass=[0 0 0]  CenterOfMassUnits=m  GraphicDiffuseColor=[0.8 0.0 0.0]  CylinderLength=0.1  CylinderLengthUnits=m  CylinderRadius=0.15  CylinderRadiusUnits=m  Density=1000  DensityUnits=kg/m^3  DoExposeReferenceFrame=on  GraphicEmissiveColor=[0.0 0.0 0.0 1.0]  ExportEntireGeometry=off  SerializedFrames=<Frames/>  MarkerShape=Sphere  MarkerSize=10  GraphicType=FromGeometry  InertiaType=Custom  Mass=RWS.m  MassUnits=kg  MomentsOfInertia=[RWS.Ir RWS.Ir RWS.Iw]  MomentsOfInertiaUnits=kg*m^2  GraphicOpacity=0.8  ProductsOfInertia=[0 0 0]  ProductsOfInertiaUnits=kg*m^2  GraphicShininess=75  GraphicSpecularColor=[0.5 0.5 0.5 1.0]  GraphicVisPropType=SimpleVisualProperties
  Frame R_RW{1..4} (4 alike) : sm_lib/Body Elements/Graphic  GraphicType=Marker  MarkerShape=Frame  MarkerSize=35  GraphicVisPropType=SimpleVisualProperties  GraphicDiffuseColor=[0.2 1.0 1.0]  GraphicSpecularColor=[0.5 0.5 0.5 1.0]  GraphicAmbientColor=[0.15 0.15 0.15 1.0]  GraphicEmissiveColor=[0.0 0.0 0.0 1.0]  GraphicShininess=75  GraphicOpacity=0.5
  Connection Port : PMIOPort  Tag=PMCPort  Side=Left
  Connection Port1 : PMIOPort  Tag=PMCPort  Port=2  Side=Left
  Connection Port2 : PMIOPort  Tag=PMCPort  Port=3  Side=Left
  Connection Port3 : PMIOPort  Tag=PMCPort  Port=4  Side=Left
  connections:
  Frame R_RW1/RConn1 -- Connection Port/RConn1 -- Cylindrical Solid/RConn1
  Cylindrical Solid1/RConn1 -- Connection Port1/RConn1 -- Frame R_RW2/RConn1
  Cylindrical Solid2/RConn1 -- Connection Port2/RConn1 -- Frame R_RW3/RConn1
  Cylindrical Solid3/RConn1 -- Connection Port3/RConn1 -- Frame R_RW4/RConn1

== system Simscape_Benchmark_SIM1/Dynamical system/WEMS + Reaction wheels/Reaction wheel Mass//inertia (balanced and unbalanced model)/RWS with disturbance harmonics ==
  note: Static imbalance
  note: Dynamic imbalance
  note: Static imbalance
  note: Dynamic imbalance
  note: Static imbalance
  note: Dynamic imbalance
  note: Static imbalance
  note: Dynamic imbalance
  note: $[r_s\,, 0\,, 0]$
  note: $m_s$
  note: $[r_d\,, 0\,, h_d]$
  note: $m_d$
  note: $[-r_d\,, 0\,, -h_d]$
  note: $m_d$
  Brick Solid{,3,6,9} (4 alike) : sm_lib/Body Elements/Brick Solid  GraphicAmbientColor=[0.15 0.15 0.15 1.0]  BasedOnType=Density  BrickDimensions=[0.01 0.01 0.01]  BrickDimensionUnits=m  CenterOfMass=[0 0 0]  CenterOfMassUnits=m  GraphicDiffuseColor=[0.5 0.5 0.5]  Density=1000  DensityUnits=kg/m^3  DoExposeReferenceFrame=on  GraphicEmissiveColor=[0.0 0.0 0.0 1.0]  ExportEntireGeometry=off  SerializedFrames=<Frames/>  MarkerShape=Sphere  MarkerSize=10  GraphicType=None  InertiaType=PointMass  Mass=RWS.m_s  MassUnits=kg  MomentsOfInertia=[1 1 1]  MomentsOfInertiaUnits=kg*m^2  GraphicOpacity=1.0  ProductsOfInertia=[0 0 0]  ProductsOfInertiaUnits=kg*m^2  GraphicShininess=75  GraphicSpecularColor=[0.5 0.5 0.5 1.0]  GraphicVisPropType=SimpleVisualProperties
  Brick Solid{1..2,4..5,7..8,10..11} (8 alike) : sm_lib/Body Elements/Brick Solid  GraphicAmbientColor=[0.15 0.15 0.15 1.0]  BasedOnType=Density  BrickDimensions=[0.01 0.01 0.01]  BrickDimensionUnits=m  CenterOfMass=[0 0 0]  CenterOfMassUnits=m  GraphicDiffuseColor=[0.5 0.5 0.5]  Density=1000  DensityUnits=kg/m^3  DoExposeReferenceFrame=on  GraphicEmissiveColor=[0.0 0.0 0.0 1.0]  ExportEntireGeometry=off  SerializedFrames=<Frames/>  MarkerShape=Sphere  MarkerSize=10  GraphicType=None  InertiaType=PointMass  Mass=RWS.m_d  MassUnits=kg  MomentsOfInertia=[1 1 1]  MomentsOfInertiaUnits=kg*m^2  GraphicOpacity=1.0  ProductsOfInertia=[0 0 0]  ProductsOfInertiaUnits=kg*m^2  GraphicShininess=75  GraphicSpecularColor=[0.5 0.5 0.5 1.0]  GraphicVisPropType=SimpleVisualProperties
  Cylindrical Solid{,1..3} (4 alike) : sm_lib/Body Elements/Cylindrical Solid  GraphicAmbientColor=[0.15 0.15 0.15 1.0]  BasedOnType=Density  CenterOfMass=[0 0 0]  CenterOfMassUnits=m  GraphicDiffuseColor=[0.5 0.5 0.5]  CylinderLength=0.1  CylinderLengthUnits=m  CylinderRadius=0.15  CylinderRadiusUnits=m  Density=1000  DensityUnits=kg/m^3  DoExposeReferenceFrame=on  GraphicEmissiveColor=[0.0 0.0 0.0 1.0]  ExportEntireGeometry=off  SerializedFrames=<Frames/>  MarkerShape=Sphere  MarkerSize=10  GraphicType=FromGeometry  InertiaType=Custom  Mass=RWS.m  MassUnits=kg  MomentsOfInertia=[RWS.Ir RWS.Ir RWS.Iw]  MomentsOfInertiaUnits=kg*m^2  GraphicOpacity=1.0  ProductsOfInertia=[0 0 0]  ProductsOfInertiaUnits=kg*m^2  GraphicShininess=75  GraphicSpecularColor=[0.5 0.5 0.5 1.0]  GraphicVisPropType=SimpleVisualProperties
  Frame R_RW1 : sm_lib/Body Elements/Graphic  GraphicType=Marker  MarkerShape=Frame  MarkerSize=45  GraphicVisPropType=SimpleVisualProperties  GraphicDiffuseColor=[0.2 1.0 1.0]  GraphicSpecularColor=[0.5 0.5 0.5 1.0]  GraphicAmbientColor=[0.15 0.15 0.15 1.0]  GraphicEmissiveColor=[0.0 0.0 0.0 1.0]  GraphicShininess=75  GraphicOpacity=1.0
  Frame R_RW2 : sm_lib/Body Elements/Graphic  GraphicType=Marker  MarkerShape=Frame  MarkerSize=25  GraphicVisPropType=SimpleVisualProperties  GraphicDiffuseColor=[0.2 1.0 1.0]  GraphicSpecularColor=[0.5 0.5 0.5 1.0]  GraphicAmbientColor=[0.15 0.15 0.15 1.0]  GraphicEmissiveColor=[0.0 0.0 0.0 1.0]  GraphicShininess=75  GraphicOpacity=1.0
  Frame R_RW3 : sm_lib/Body Elements/Graphic  GraphicType=Marker  MarkerShape=Frame  MarkerSize=50  GraphicVisPropType=SimpleVisualProperties  GraphicDiffuseColor=[0.2 1.0 1.0]  GraphicSpecularColor=[0.5 0.5 0.5 1.0]  GraphicAmbientColor=[0.15 0.15 0.15 1.0]  GraphicEmissiveColor=[0.0 0.0 0.0 1.0]  GraphicShininess=75  GraphicOpacity=1.0
  Frame R_RW4 : sm_lib/Body Elements/Graphic  GraphicType=Marker  MarkerShape=Frame  MarkerSize=25  GraphicVisPropType=SimpleVisualProperties  GraphicDiffuseColor=[0.2 1.0 1.0]  GraphicSpecularColor=[0.5 0.5 0.5 1.0]  GraphicAmbientColor=[0.15 0.15 0.15 1.0]  GraphicEmissiveColor=[0.0 0.0 0.0 1.0]  GraphicShininess=75  GraphicOpacity=1.0
  Rigid Transform{,2,5,9} (4 alike) : sm_lib/Frames and Transforms/Rigid Transform  TranslationMethod=Cartesian  TranslationStandardOffset=0  TranslationLengthUnit=m  TranslationStandardAxis=+Z  TranslationCartesianOffset=[RWS.r_d 0 RWS.h_d]  TranslationROffset=0  TranslationROffsetUnits=m  TranslationZOffset=0  TranslationZOffsetUnits=m  TranslationThetaOffset=0  TranslationThetaOffsetUnits=deg  RotationMethod=None  RotationAngleUnits=deg  RotationStandardAxis=+Z  RotationAngle=0.0  RotationArbitraryAxis=[0 0 1]  FollAlignAxisA=+X  BaseAlignAxisA=+Y  FollAlignAxisB=+Y  BaseAlignAxisB=+Z  RotationSequenceAxes=FollowerAxes  RotationSequence=XYX  RotationSequenceAngles=[0 0 0]  RotationSequenceAnglesUnits=deg  RotationMatrix=[1 0 0; 0 1 0; 0 0 1]
  Rigid Transform{1,3,7,10} (4 alike) : sm_lib/Frames and Transforms/Rigid Transform  TranslationMethod=Cartesian  TranslationStandardOffset=0  TranslationLengthUnit=m  TranslationStandardAxis=+Z  TranslationCartesianOffset=[-RWS.r_d 0 -RWS.h_d]  TranslationROffset=0  TranslationROffsetUnits=m  TranslationZOffset=0  TranslationZOffsetUnits=m  TranslationThetaOffset=0  TranslationThetaOffsetUnits=deg  RotationMethod=None  RotationAngleUnits=deg  RotationStandardAxis=+Z  RotationAngle=0.0  RotationArbitraryAxis=[0 0 1]  FollAlignAxisA=+X  BaseAlignAxisA=+Y  FollAlignAxisB=+Y  BaseAlignAxisB=+Z  RotationSequenceAxes=FollowerAxes  RotationSequence=XYX  RotationSequenceAngles=[0 0 0]  RotationSequenceAnglesUnits=deg  RotationMatrix=[1 0 0; 0 1 0; 0 0 1]
  Rigid Transform{4,6,8,11} (4 alike) : sm_lib/Frames and Transforms/Rigid Transform  TranslationMethod=Cartesian  TranslationStandardOffset=0  TranslationLengthUnit=m  TranslationStandardAxis=+Z  TranslationCartesianOffset=[RWS.r_s 0 0]  TranslationROffset=0  TranslationROffsetUnits=m  TranslationZOffset=0  TranslationZOffsetUnits=m  TranslationThetaOffset=0  TranslationThetaOffsetUnits=deg  RotationMethod=None  RotationAngleUnits=deg  RotationStandardAxis=+Z  RotationAngle=0.0  RotationArbitraryAxis=[0 0 1]  FollAlignAxisA=+X  BaseAlignAxisA=+Y  FollAlignAxisB=+Y  BaseAlignAxisB=+Z  RotationSequenceAxes=FollowerAxes  RotationSequence=XYX  RotationSequenceAngles=[0 0 0]  RotationSequenceAnglesUnits=deg  RotationMatrix=[1 0 0; 0 1 0; 0 0 1]
  Connection Port : PMIOPort  Tag=PMCPort  Side=Left
  Connection Port1 : PMIOPort  Tag=PMCPort  Port=2  Side=Left
  Connection Port2 : PMIOPort  Tag=PMCPort  Port=3  Side=Left
  Connection Port3 : PMIOPort  Tag=PMCPort  Port=4  Side=Left
  connections:
  Brick Solid1/RConn1 -- Rigid Transform/RConn1
  Rigid Transform1/RConn1 -- Brick Solid2/RConn1
  Rigid Transform6/RConn1 -- Brick Solid/RConn1
  Rigid Transform1/LConn1 -- Frame R_RW1/RConn1 -- Connection Port/RConn1 -- Cylindrical Solid/RConn1 -- Rigid Transform6/LConn1 -- Rigid Transform/LConn1
  Rigid Transform2/LConn1 -- Rigid Transform4/LConn1 -- Rigid Transform3/LConn1 -- Connection Port1/RConn1 -- Cylindrical Solid1/RConn1 -- Frame R_RW2/RConn1
  Rigid Transform5/LConn1 -- Rigid Transform8/LConn1 -- Rigid Transform7/LConn1 -- Connection Port2/RConn1 -- Cylindrical Solid2/RConn1 -- Frame R_RW3/RConn1
  Rigid Transform9/LConn1 -- Frame R_RW4/RConn1 -- Cylindrical Solid3/RConn1 -- Connection Port3/RConn1 -- Rigid Transform11/LConn1 -- Rigid Transform10/LConn1
  Rigid Transform3/RConn1 -- Brick Solid5/RConn1
  Brick Solid4/RConn1 -- Rigid Transform2/RConn1
  Rigid Transform4/RConn1 -- Brick Solid3/RConn1
  Rigid Transform8/RConn1 -- Brick Solid6/RConn1
  Rigid Transform7/RConn1 -- Brick Solid8/RConn1
  Brick Solid7/RConn1 -- Rigid Transform5/RConn1
  Rigid Transform10/RConn1 -- Brick Solid11/RConn1
  Brick Solid10/RConn1 -- Rigid Transform9/RConn1
  Rigid Transform11/RConn1 -- Brick Solid9/RConn1

== system Simscape_Benchmark_SIM1/Dynamical system/Payload System (Telescope structure, FSM, PMA system, Isolator)/Integration/Quaternion Integration2/Subsystem ==
  q_4 : Inport
  om : Inport  Port=2
  Cross Product : vrlib/Utilities/Cross Product
  Demux : Demux  Outputs=[1 3]
  Dot Product : DotProduct  InputSameDT=on  OutDataTypeStr=Inherit: Inherit via internal rule
  Gain : Gain  Gain=0.5
  Gain1 : Gain  Gain=-1
  Gain2 : Gain  Gain=-1
  Mux : Mux  Inputs=[1,3]
  Product : Product
  Sum : Sum  Inputs=|+-
  Out1 : Outport
  wires:
  Gain/1 -> Out1/1
  Mux/1 -> Gain/1
  Demux/1 -> Product/2  "q0"
  Demux/2 -> Cross Product/2, Dot Product/2  "q"
  q_4/1 -> Demux/1
  Dot Product/1 -> Gain1/1
  om/1 -> Cross Product/1, Product/1, Dot Product/1
  Gain1/1 -> Mux/1
  Sum/1 -> Mux/2
  Product/1 -> Sum/1
  Cross Product/1 -> Gain2/1
  Gain2/1 -> Sum/2

== system Simscape_Benchmark_SIM1/Dynamical system/Payload System (Telescope structure, FSM, PMA system, Isolator)/Integration 1/Quaternion Integration1/Subsystem ==
  q_4 : Inport
  om : Inport  Port=2
  Cross Product : vrlib/Utilities/Cross Product
  Demux : Demux  Outputs=[1 3]
  Dot Product : DotProduct  InputSameDT=on  OutDataTypeStr=Inherit: Inherit via internal rule
  Gain : Gain  Gain=0.5
  Gain1 : Gain  Gain=-1
  Gain2 : Gain  Gain=-1
  Mux : Mux  Inputs=[1,3]
  Product : Product
  Sum : Sum  Inputs=|+-
  Out1 : Outport
  wires:
  Gain/1 -> Out1/1
  Mux/1 -> Gain/1
  Demux/1 -> Product/2  "q0"
  Demux/2 -> Cross Product/2, Dot Product/2  "q"
  q_4/1 -> Demux/1
  Dot Product/1 -> Gain1/1
  om/1 -> Cross Product/1, Product/1, Dot Product/1
  Gain1/1 -> Mux/1
  Sum/1 -> Mux/2
  Product/1 -> Sum/1
  Cross Product/1 -> Gain2/1
  Gain2/1 -> Sum/2

== system Simscape_Benchmark_SIM1/Dynamical system/WEMS + Reaction wheels/RW saturation and friction model/Saturations +  friction model/RW friction model ==
  Trq_cmd_rw : Inport
  Friction model (torque) : Subsystem
  Mux : Mux
  Rate Transition : RateTransition  OutPortSampleTime=Model.ACS_sampling.Ts
  Torque_RW : Outport
  RW_TRQfriction : Outport  Port=2  VectorParamsAs1DForOutWhenUnconnected=off
  tag scope: RW_Friction=global
  wires:
  [RW4_speed] -> Mux/4
  Mux/1 -> Rate Transition/1
  Trq_cmd_rw/1 -> Friction model (torque)/2(motor cmd trq (Nm))
  Friction model (torque)/2(Torque_friction) -> [RW_Friction], RW_TRQfriction/1  "rw_Trqfriction"
  [RW2_speed] -> Mux/2
  [RW3_speed] -> Mux/3
  [RW1_speed] -> Mux/1
  Rate Transition/1 -> Friction model (torque)/1(rw_speed (rad/s))
  Friction model (torque)/1(Torque_total) -> Torque_RW/1

== system Simscape_Benchmark_SIM1/Dynamical system/WEMS + Reaction wheels/RW saturation and friction model/Saturations + friction model + friction spikes/RW friction model ==
  Trq_cmd_rw : Inport
  Friction model (torque)1 : Subsystem
  Mux : Mux
  Rate Transition : RateTransition  OutPortSampleTime=Model.ACS_sampling.Ts
  Torque_RW : Outport
  RW_TRQfriction : Outport  Port=2  VectorParamsAs1DForOutWhenUnconnected=off
  sign_omega : Outport  Port=3
  tag scope: RW_Friction=global
  wires:
  [RW4_speed] -> Mux/4
  Mux/1 -> Rate Transition/1
  Trq_cmd_rw/1 -> Friction model (torque)1/2(motor cmd trq (Nm))
  Friction model (torque)1/2(Torque_friction) -> [RW_Friction], RW_TRQfriction/1  "rw_Trqfriction"
  [RW2_speed] -> Mux/2
  Friction model (torque)1/1(Torque_total) -> Torque_RW/1
  [RW3_speed] -> Mux/3
  [RW1_speed] -> Mux/1
  Rate Transition/1 -> Friction model (torque)1/1(rw_speed (rad/s))
  Friction model (torque)1/3(sign_omega) -> sign_omega/1

== system Simscape_Benchmark_SIM1/Dynamical system/WEMS + Reaction wheels/RW saturation and friction model/Saturations + friction model + friction spikes/Spike generation RW1 ==
  note: The condition above triggers the calculation of the spike level and the repetition time.
      | While the time_counter < Rep_time the trigger is not activated. As soon as the condition is met. The logical operator {>} activates the trigger_spike subsystem and resets the counter.
  note: The function counts how many times the {>} is activated. The output values is also used in the selection of the first repetition time since this is not initialized with trigger_spike.
  note: This part is done to avoid having a first spike always at t=t_duration of spike (which is 20 sec in this case)...so we have a trigger that for the first time (when the subsystem that computes the spike repetition time has still not been triggered) choose the time of the first initial spike.... the other time will be the t_duration that sums yp with the spike repetition time
  Constant16 : Constant  Value=RWS.spike.duration
  Constant17 : Constant  Value=0  SampleTime=Inf
  Constant18 : Constant  Value=RWS.spike.repetition.w1_Initialization  SampleTime=Inf
  Constant4 : Constant  Value=0  SampleTime=Inf
  Couter with reset function given by a condition : Subsystem
  Gain4 : Gain  Gain=10
  Gain5 : Gain  Gain=1/10
  Memory12 : Memory  InheritSampleTime=on
  Memory13 : Memory  InheritSampleTime=on
  Memory14 : Memory
  Memory15 : Memory  InheritSampleTime=on
  Relational Operator3 : RelationalOperator  Operator=>  OutDataTypeStr=boolean  RndMeth=Simplest
  Round2 : Rounding  Operator=round
  Scope{5,15,20..22} (5 alike) : Scope
  Scope23 : Scope  NumInputPorts=3
  Set_spike_duration : MATLAB Function  TreatAsAtomicUnit=on
  Sum2 : Sum  Inputs=|++
  Sum8 : Sum  Inputs=|++
  Switch3 : Switch  Criteria=u2 > Threshold  Threshold=RWS.spike.duration/Model.ACS_sampling.Ts
  Switch7 : Switch  Criteria=u2 > Threshold  Threshold=1
  Trigger_spike : Subsystem  TreatAsAtomicUnit=on
  Triggered_spikes_counter : Subsystem  TreatAsAtomicUnit=on
  Out1 : Outport
  wires:
  Constant16/1 -> Switch7/1
  Sum8/1 -> Relational Operator3/2, Scope20/1
  Gain5/1 -> Switch7/3
  Set_spike_duration/1(y) -> Switch3/2, Memory15/1
  Relational Operator3/1 -> Scope23/2, Triggered_spikes_counter/Trigger, Couter with reset function given by a condition/1(In1), Trigger_spike/Trigger
  Constant18/1 -> Gain4/1
  Sum2/1 -> Set_spike_duration/3(counter)
  Constant4/1 -> Sum2/1
  Round2/1 -> Gain5/1
  Memory12/1 -> Set_spike_duration/2(uk_1)
  Memory13/1 -> Sum8/1
  Trigger_spike/1(Spike_level) -> Set_spike_duration/1(uk), Switch3/3, Memory12/1, Scope5/1, Scope23/1
  Memory14/1 -> Sum8/2
  Trigger_spike/2(Rep_time) -> Memory13/1
  Switch3/1 -> Out1/1, Scope21/1  "Spike(t)"
  Constant17/1 -> Switch3/1
  Memory15/1 -> Sum2/2
  Triggered_spikes_counter/1(Out1) -> Scope15/1, Switch7/2
  Gain4/1 -> Round2/1
  Couter with reset function given by a condition/1(Time_counter) -> Relational Operator3/1, Scope23/3
  Switch7/1 -> Scope22/1, Memory14/1
